simulink model "DSMS_sim"  (R2019b)
settings: Solver=ode4  StartTime=0.0  StopTime=Te  FixedStep=Ts  RelTol=1e-3
values from neighbouring files (symbols this model uses):
  A = [ 0 1 ; -c/m -d/m ]    [DSMS_visu.m]    (also in init_DSMS.m)
  B = [ 0 1/m ]'    [DSMS_visu.m]    (also in init_DSMS.m)
  c = 20    [init_DSMS.m]
  C = diag([1, 1])    [DSMS_visu.m]    (also in init_DSMS.m)
  d = 10    [init_DSMS.m]
  D = zeros(size(C,1),size(B,2))    [DSMS_visu.m]    (also in init_DSMS.m)
  K = [Kp Kd]    [init_DSMS.m]
  m = 10    [init_DSMS.m]
  params = [m c d]    [init_DSMS.m]
  x1_ic = zeros(2,1)    [init_DSMS.m]
settings Model: Creator=Jakob  LastModifiedBy=Jakob

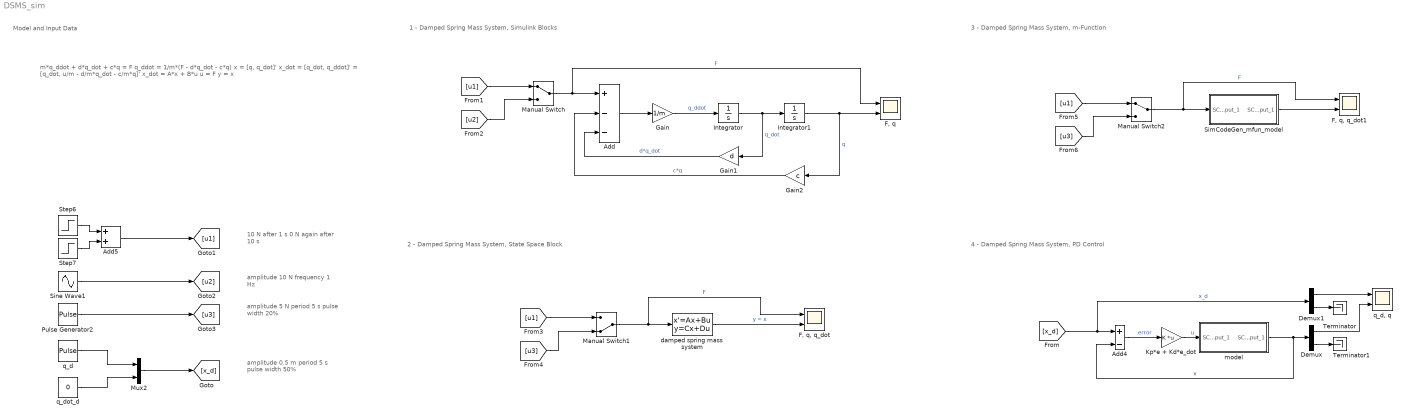
== system DSMS_sim ==
  note: 10 N after 1 s
      |   0 N again after 10 s
  note: Model and Input Data
  note: 2 - Damped Spring Mass System, State Space Block
  note: 1 - Damped Spring Mass System, Simulink Blocks
  note: 4 - Damped Spring Mass System, PD Control
  note: 3 - Damped Spring Mass System, m-Function
  note: amplitude 10 N
      | frequency 1 Hz
  note: amplitude 5 N
      | period 5 s
      | pulse width 20%
  note: amplitude 0.5 m
      | period 5 s
      | pulse width 50%
  note: m*q_ddot + d*q_dot + c*q = F
      | q_ddot = 1/m*(F - d*q_dot - c*q)
      |
      | x = [q, q_dot]'
      | x_dot = [q_dot, q_ddot]' = [q_dot, u/m - d/m*q_dot - c/m*q]'
      |
      | x_dot = A*x + B*u
      | u = F
      | y = x
  Add : Sum  Inputs=+--
  Add4 : Sum  Inputs=+-
  Add5 : Sum
  Demux : Demux  Outputs=2
  Demux1 : Demux  Outputs=2
  "F, q" : Scope  NumInputPorts=2
  "F, q, q_dot" : Scope  NumInputPorts=2
  "F, q, q_dot1" : Scope  NumInputPorts=2
  Gain : Gain  Gain=1/m
  Gain1 : Gain  Gain=d
  Gain2 : Gain  Gain=c
  Integrator : Integrator
  Integrator1 : Integrator
  Kp*e + Kd*e_dot : Gain  Gain=K  Multiplication=Matrix(K*u)
  Manual Switch : ManualSwitch
  Manual Switch1 : ManualSwitch  CurrentSetting=0
  Manual Switch2 : ManualSwitch
  Mux2 : Mux  Inputs=2
  Pulse Generator2 : DiscretePulseGenerator  PulseType=Time based  Amplitude=5  Period=5  PulseWidth=20
  SimCodeGen_mfun_model : Subsystem  mask{SC_param_0=params, SC_x1_ic=x1_ic}
      mask prompts: SC_param_0 "params"
      mask Display:
      | port_label('input', 1, 'u');
      | port_label('output', 1, 'x_ss');
  Sine Wave1 : Sin  Amplitude=10  SampleTime=0
  Step6 : Step  After=10  SampleTime=0
  Step7 : Step  Time=10  After=-10  SampleTime=0
  Terminator : Terminator
  Terminator1 : Terminator
  damped spring mass system : StateSpace  A=A  B=B  C=C  D=D  InitialCondition=[0;0]
  model : Subsystem  mask{SC_param_0=params, SC_x1_ic=x1_ic}
      mask prompts: SC_param_0 "params"
      mask Display:
      | port_label('input', 1, 'u');
      | port_label('output', 1, 'x_ss');
  q_d : DiscretePulseGenerator  PulseType=Time based  Amplitude=0.5  Period=5  PulseWidth=50
  "q_d, q" : Scope  NumInputPorts=2
  q_dot_d : Constant  Value=0
  wires:
  Add/1 -> Gain/1
  Gain/1 -> Integrator/1  "q_ddot"
  Integrator/1 -> Gain1/1, Integrator1/1  "q_dot"
  Integrator1/1 -> "F, q"/2, Gain2/1  "q"
  Gain1/1 -> Add/3  "d*q_dot"
  Gain2/1 -> Add/2  "c*q"
  Manual Switch/1 -> "F, q"/1, Add/1  "F"
  [u1] -> Manual Switch/1
  [u2] -> Manual Switch/2
  [u1] -> Manual Switch1/1
  damped spring mass system/1 -> "F, q, q_dot"/2  "y = x"
  Manual Switch1/1 -> "F, q, q_dot"/1, damped spring mass system/1  "F"
  [u3] -> Manual Switch1/2
  SimCodeGen_mfun_model/1(SC_output_1) -> "F, q, q_dot1"/2
  Manual Switch2/1 -> SimCodeGen_mfun_model/1(SC_input_1), "F, q, q_dot1"/1  "F"
  q_dot_d/1 -> Mux2/2
  q_d/1 -> Mux2/1
  Demux/2 -> Terminator1/1
  Demux/1 -> "q_d, q"/2
  Demux1/2 -> Terminator/1
  Demux1/1 -> "q_d, q"/1
  Kp*e + Kd*e_dot/1 -> model/1(SC_input_1)  "u"
  model/1(SC_output_1) -> Demux/1, Add4/2  "x"
  Add4/1 -> Kp*e + Kd*e_dot/1  "error"
  [x_d] -> Demux1/1, Add4/1  "x_d"
  Step6/1 -> Add5/1
  Step7/1 -> Add5/2
  Add5/1 -> [u1]
  Sine Wave1/1 -> [u2]
  Pulse Generator2/1 -> [u3]
  [u1] -> Manual Switch2/1
  [u3] -> Manual Switch2/2
  Mux2/1 -> [x_d]

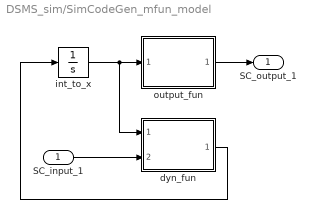
== system DSMS_sim/SimCodeGen_mfun_model ==
  SC_input_1 : Inport
  dyn_fun : MATLAB Function  TreatAsAtomicUnit=on
  int_to_x : Integrator  InitialCondition=[SC_x1_ic]
  output_fun : MATLAB Function  TreatAsAtomicUnit=on
  SC_output_1 : Outport
  wires:
  output_fun/1(SC_output_0) -> SC_output_1/1
  dyn_fun/1(SC_state_dot) -> int_to_x/1
  SC_input_1/1 -> dyn_fun/2(SC_input_0)
  int_to_x/1 -> output_fun/1(SC_state), dyn_fun/1(SC_state)

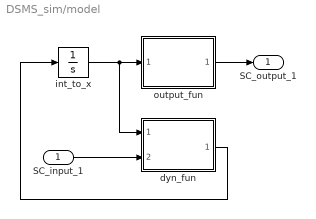
== system DSMS_sim/model ==
  SC_input_1 : Inport
  dyn_fun : MATLAB Function  TreatAsAtomicUnit=on
  int_to_x : Integrator  InitialCondition=[SC_x1_ic]
  output_fun : MATLAB Function  TreatAsAtomicUnit=on
  SC_output_1 : Outport
  wires:
  int_to_x/1 -> dyn_fun/1(SC_state), output_fun/1(SC_state)
  SC_input_1/1 -> dyn_fun/2(SC_input_0)
  dyn_fun/1(SC_state_dot) -> int_to_x/1
  output_fun/1(SC_output_0) -> SC_output_1/1

== matlab function DSMS_sim/SimCodeGen_mfun_model/output_fun ==
  data: SC_state input size=[2]; SC_output_0 output size=[2]; SC_param_0 parameter size=[3]
function SC_output_0  = y_fun(SC_state, SC_param_0)
    SC_output_0 = zeros(2,1);
    SC_state_x_0 = SC_state(1:2);
    SC_output_0(1) = SC_state_x_0(1);
    SC_output_0(2) = SC_state_x_0(2);
end

== matlab function DSMS_sim/SimCodeGen_mfun_model/dyn_fun ==
  data: SC_state input size=[2]; SC_state_dot output size=[2]; SC_input_0 input size=[1]; SC_param_0 parameter
function SC_state_dot  = dyn_fun(SC_state, SC_input_0, SC_param_0)
    SC_state_dot = zeros(2, 1);
    SC_state_x_0 = SC_state(1:2);
    SC_eval = zeros(2,1);
    SC_eval(1) = SC_state_x_0(2);
    SC_eval(2) = -(SC_eval(1) * SC_param_0(3) + SC_param_0(2) * SC_state_x_0(1) - SC_input_0(1)) / SC_param_0(1);
    SC_state_dot(1:2) = SC_eval(1:2);
end

== matlab function DSMS_sim/model/dyn_fun ==
  data: SC_state input size=[2]; SC_state_dot output size=[2]; SC_input_0 input size=[1]; SC_param_0 parameter
function SC_state_dot  = dyn_fun(SC_state, SC_input_0, SC_param_0)
    SC_state_dot = zeros(2, 1);
    SC_state_x_0 = SC_state(1:2);
    SC_eval = zeros(2,1);
    SC_eval(1) = SC_state_x_0(2);
    SC_eval(2) = -(SC_eval(1) * SC_param_0(3) + SC_param_0(2) * SC_state_x_0(1) - SC_input_0(1)) / SC_param_0(1);
    SC_state_dot(1:2) = SC_eval(1:2);
end

== matlab function DSMS_sim/model/output_fun ==
  data: SC_state input size=[2]; SC_output_0 output size=[2]; SC_param_0 parameter size=[3]
function SC_output_0  = y_fun(SC_state, SC_param_0)
    SC_output_0 = zeros(2,1);
    SC_state_x_0 = SC_state(1:2);
    SC_output_0(1) = SC_state_x_0(1);
    SC_output_0(2) = SC_state_x_0(2);
end
